simulink model "ppm"  (R2018a)
settings: Solver=VariableStepAuto  StartTime=0.0  StopTime=10.0  RelTol=1e-3
libraries: simulink_extras x1
settings Model: Creator=shahb  LastModifiedBy=shahb

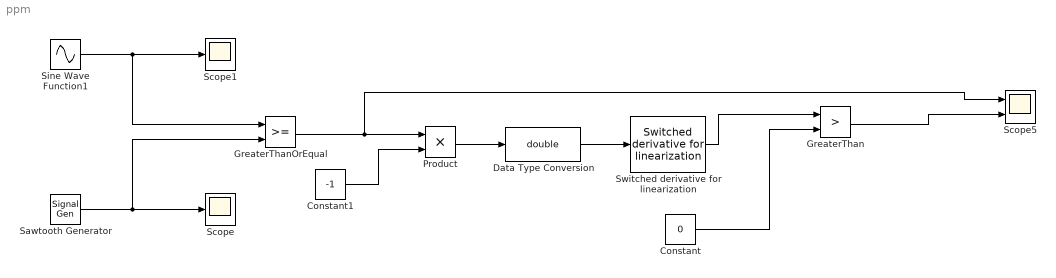
== system ppm ==
  Constant : Constant  Value=0
  Constant1 : Constant  Value=-1
  Data Type Conversion : DataTypeConversion  OutDataTypeStr=double
  GreaterThan : RelationalOperator  Operator=>  OutDataTypeStr=boolean  RndMeth=Simplest
  GreaterThanOrEqual : RelationalOperator  OutDataTypeStr=boolean  RndMeth=Simplest
  Product : Product
  Sawtooth Generator : SignalGenerator  WaveForm=sawtooth  Amplitude=5  Frequency=10  Units=rad/sec
  Scope : Scope
  Scope1 : Scope
  Scope5 : Scope  NumInputPorts=2
  Sine Wave Function1 : Sin  Frequency=5  SampleTime=0
  Switched derivative for linearization : simulink_extras/Linearization/Switched derivative for linearization  switchVal=0  derivConst=100
      settings: SourceProductName=Simulink  SourceProductBaseCode=SL
  wires:
  Sawtooth Generator/1 -> Scope/1, GreaterThanOrEqual/2
  Data Type Conversion/1 -> Switched derivative for linearization/1
  GreaterThanOrEqual/1 -> Scope5/1, Product/1
  Sine Wave Function1/1 -> GreaterThanOrEqual/1, Scope1/1
  Constant1/1 -> Product/2
  Product/1 -> Data Type Conversion/1
  Switched derivative for linearization/1 -> GreaterThan/1
  Constant/1 -> GreaterThan/2
  GreaterThan/1 -> Scope5/2
